simulink subsystem "AUVPlant"  (R2020a)
settings: Solver=VariableStepAuto  StartTime=0.0  StopTime=10.0  RelTol=1e-3
undefined symbols (not defined in the file or in its folder): dMaxX, dMaxY, dMinX, dMinY, dSeedX, dSeedY, dts, N, PWM, T200, tmax, tmin, waPhi, waPsi, waTheta, waX, waY, waZ, wfPhi, wfPsi, wfTheta, wfX, wfY, wfZ, wpPhi, wpPsi, wpTheta, wpX, wpY, wpZ
libraries: simulink x2
settings Model: Creator=lamarre  LastModifiedBy=lamarre

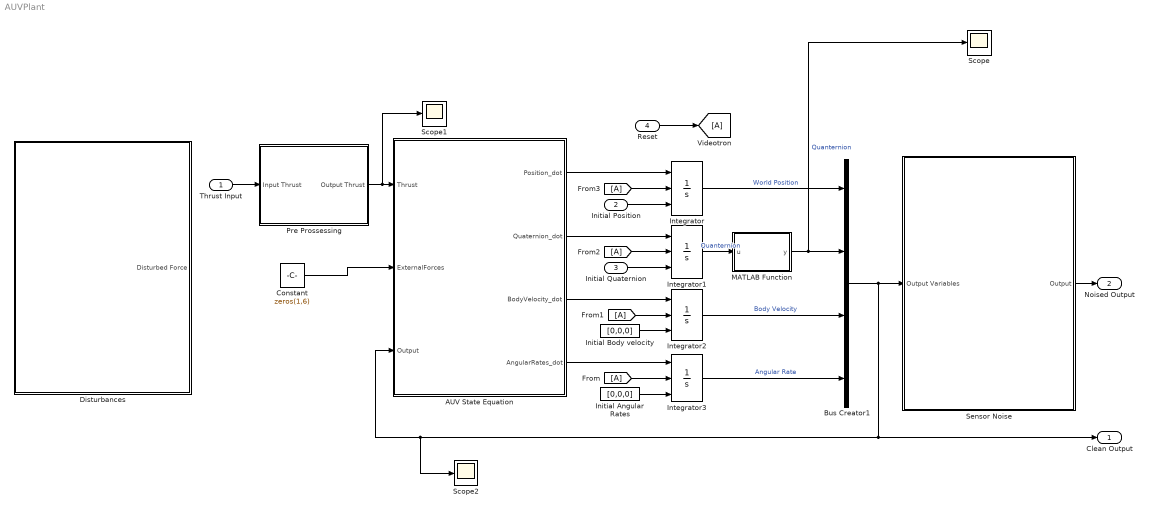
== system AUVPlant ==
  Thrust Input : Inport
  Initial Position : Inport  Port=2
  Initial Quaternion : Inport  Port=3
  Reset : Inport  Port=4
  AUV State Equation : MATLAB Function  TreatAsAtomicUnit=on  SystemSampleTime=.005
  Bus Creator1 : BusCreator  Inputs=4
  Constant : Constant  Value=zeros(1,6)
  Disturbances : Subsystem
  Initial Angular Rates : Constant  Value=[0,0,0]
  "Initial Body velocity " : Constant  Value=[0,0,0]
  Integrator : Integrator  ExternalReset=rising  InitialConditionSource=external  InitialCondition=[0,0,1]
  Integrator1 : Integrator  ExternalReset=rising  InitialConditionSource=external  InitialCondition=[1,0,0,0]
  Integrator2 : Integrator  ExternalReset=rising  InitialConditionSource=external  InitialCondition=[0,0,0]
  Integrator3 : Integrator  ExternalReset=rising  InitialConditionSource=external  InitialCondition=[0,0,0]
  MATLAB Function : MATLAB Function  TreatAsAtomicUnit=on
  Pre Prossessing : Subsystem
  Scope : Scope
  Scope1 : Scope
  Scope2 : Scope
  Sensor Noise : Subsystem
  Clean Output : Outport
  Noised Output : Outport  Port=2
  wires:
  "Initial Body velocity "/1 -> Integrator2/3
  AUV State Equation/2(Quaternion_dot) -> Integrator1/1
  Integrator/1 -> Bus Creator1/1  "World Position"
  Integrator2/1 -> Bus Creator1/3  "Body Velocity"
  AUV State Equation/1(Position_dot) -> Integrator/1
  Initial Angular Rates/1 -> Integrator3/3
  Thrust Input/1 -> Pre Prossessing/1(Input Thrust)
  AUV State Equation/4(AngularRates_dot) -> Integrator3/1
  Integrator3/1 -> Bus Creator1/4  "Angular Rate"
  Initial Quaternion/1 -> Integrator1/3
  AUV State Equation/3(BodyVelocity_dot) -> Integrator2/1
  [A] -> Integrator3/2
  [A] -> Integrator2/2
  [A] -> Integrator1/2
  [A] -> Integrator/2
  Initial Position/1 -> Integrator/3
  Reset/1 -> [A]
  Sensor Noise/1(Output) -> Noised Output/1
  Pre Prossessing/1(Output Thrust) -> AUV State Equation/1(Thrust), Scope1/1
  Bus Creator1/1 -> AUV State Equation/3(Output), Scope2/1, Clean Output/1, Sensor Noise/1(Output Variables)
  Integrator1/1 -> MATLAB Function/1(u)  "Quanternion"
  Constant/1 -> AUV State Equation/2(ExternalForces)
  MATLAB Function/1(y) -> Bus Creator1/2, Scope/1  "Quanternion"

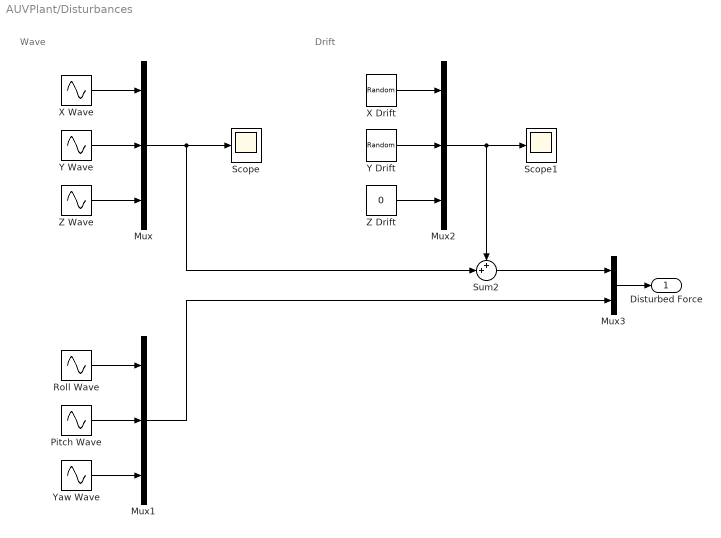
== system AUVPlant/Disturbances ==
  note: Drift
  note: Wave
  Mux : Mux  Inputs=3
  Mux1 : Mux  Inputs=3
  Mux2 : Mux  Inputs=3
  Mux3 : Mux  Inputs=2
  Pitch Wave : Sin  Amplitude=waTheta  Frequency=wfTheta  Phase=wpTheta  SampleTime=0
  Roll Wave : Sin  Amplitude=waPhi  Frequency=wfPhi  Phase=wpPhi  SampleTime=0
  Scope : Scope
  Scope1 : Scope
  Sum2 : Sum  Inputs=++|
  X Drift : UniformRandomNumber  Minimum=dMinX  Maximum=dMaxX  Seed=dSeedX  SampleTime=dts
  X Wave : Sin  Amplitude=waX  Frequency=wfX  Phase=wpX  SampleTime=0
  Y Drift : UniformRandomNumber  Minimum=dMinY  Maximum=dMaxY  Seed=dSeedY  SampleTime=dts
  Y Wave : Sin  Amplitude=waY  Frequency=wfY  Phase=wpY  SampleTime=0
  Yaw Wave : Sin  Amplitude=waPsi  Frequency=wfPsi  Phase=wpPsi  SampleTime=0
  Z Drift : Constant  Value=0
  Z Wave : Sin  Amplitude=waZ  Frequency=wfZ  Phase=wpZ  SampleTime=0
  Disturbed Force : Outport
  wires:
  Roll Wave/1 -> Mux1/1
  Pitch Wave/1 -> Mux1/2
  Mux3/1 -> Disturbed Force/1
  Sum2/1 -> Mux3/1
  X Wave/1 -> Mux/1
  Y Wave/1 -> Mux/2
  Z Wave/1 -> Mux/3
  Yaw Wave/1 -> Mux1/3
  Mux1/1 -> Mux3/2
  Mux2/1 -> Scope1/1, Sum2/1
  X Drift/1 -> Mux2/1
  Y Drift/1 -> Mux2/2
  Mux/1 -> Sum2/2, Scope/1
  Z Drift/1 -> Mux2/3

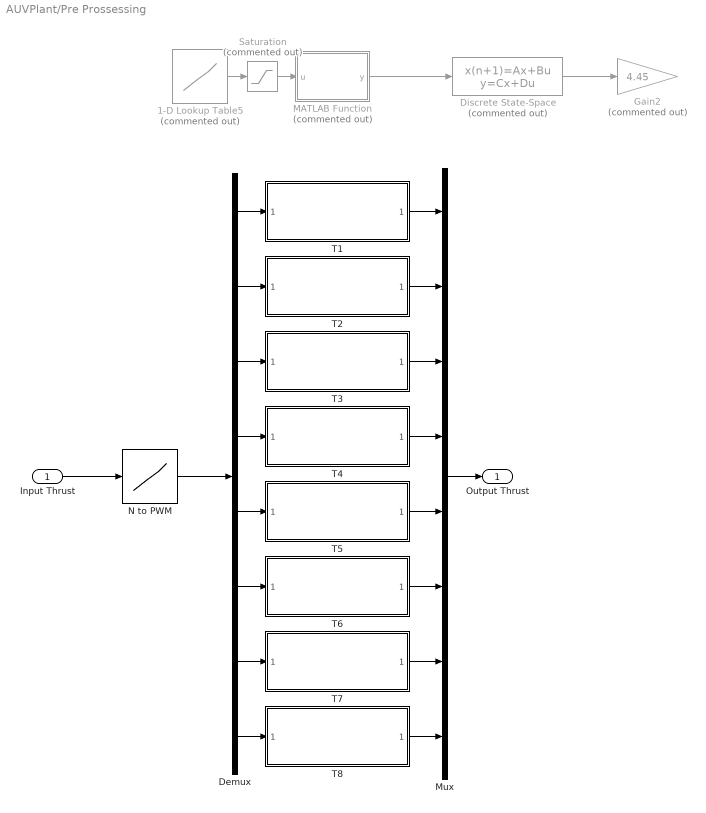
== system AUVPlant/Pre Prossessing ==
  Input Thrust : Inport
  1-D Lookup Table5 : Lookup_n-D  Commented=on  NumberOfTableDimensions=1  BreakpointsForDimension1=N  Table=PWM  InterpMethod=Nearest  InternalRulePriority=Speed  RndMeth=Simplest  InputSameDT=on
  Demux : Demux  Outputs=8
  Discrete State-Space : DiscreteStateSpace  Commented=on  A=T200.A  B=T200.B  C=T200.C  D=T200.D  SampleTime=T200.Ts
  Gain2 : Gain  Commented=on  Gain=4.45
  MATLAB Function : MATLAB Function  Commented=on  TreatAsAtomicUnit=on
  Mux : Mux  Inputs=8
  N to PWM : Lookup_n-D  NumberOfTableDimensions=1  BreakpointsForDimension1=PWM  Table=N  InterpMethod=Nearest  ExtrapMethod=Clip  InternalRulePriority=Speed  RndMeth=Simplest  InputSameDT=on
  Saturation : Saturate  Commented=on  UpperLimit=tmax  LowerLimit=tmin  LinearizeAsGain=off  ZeroCross=off
  T{1..8} (8 alike) : Subsystem  ReferencedSubsystem=ThrusterModel
  Output Thrust : Outport
  wires:
  Input Thrust/1 -> N to PWM/1
  N to PWM/1 -> Demux/1
  Saturation/1 -> MATLAB Function/1(u)
  1-D Lookup Table5/1 -> Saturation/1
  Discrete State-Space/1 -> Gain2/1
  MATLAB Function/1(y) -> Discrete State-Space/1
  Demux/1 -> T1/1
  Demux/2 -> T2/1
  Demux/3 -> T3/1
  Demux/4 -> T4/1
  Demux/5 -> T5/1
  Demux/6 -> T6/1
  Demux/8 -> T8/1
  Demux/7 -> T7/1
  T1/1 -> Mux/1
  T2/1 -> Mux/2
  T3/1 -> Mux/3
  T4/1 -> Mux/4
  T5/1 -> Mux/5
  T6/1 -> Mux/6
  T7/1 -> Mux/7
  T8/1 -> Mux/8
  Mux/1 -> Output Thrust/1

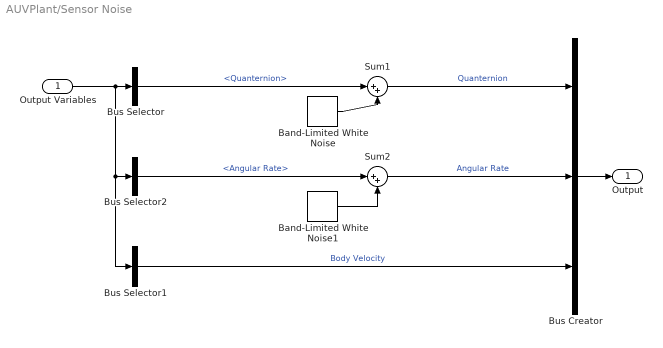
== system AUVPlant/Sensor Noise ==
  Output Variables : Inport
  Band-Limited White Noise : simulink/Sources/Band-Limited White Noise  Cov=[0.00000000025]  Ts=1/100  seed=[23341]
  Band-Limited White Noise1 : simulink/Sources/Band-Limited White Noise  Cov=[0.0000000004]  Ts=1/100  seed=[23341]
  Bus Creator : BusCreator  Inputs=3
  Bus Selector : BusSelector  OutputSignals=Quanternion
  Bus Selector1 : BusSelector  OutputSignals=Body Velocity  OutputAsBus=on
  Bus Selector2 : BusSelector  OutputSignals=Angular Rate
  Sum1 : Sum  Inputs=|++
  Sum2 : Sum  Inputs=|++
  Output : Outport
  wires:
  Sum2/1 -> Bus Creator/2  "Angular Rate"
  Sum1/1 -> Bus Creator/1  "Quanternion"
  Band-Limited White Noise1/1 -> Sum2/2
  Bus Selector2/1 -> Sum2/1  "<Angular Rate>"
  Bus Creator/1 -> Output/1
  Bus Selector1/1 -> Bus Creator/3  "Body Velocity"
  Bus Selector/1 -> Sum1/1  "<Quanternion>"
  Output Variables/1 -> Bus Selector/1, Bus Selector1/1, Bus Selector2/1
  Band-Limited White Noise/1 -> Sum1/2

== matlab function AUVPlant/MATLAB Function ==
  data: u input size=4; y output size=4
function y = Normalize(u)

d=norm(u);
y = u/d;

== matlab function AUVPlant/AUV State Equation ==
  data: Thrust input; ExternalForces input; Output input; Position_dot output size=3; Quaternion_dot output size=4; BodyVelocity_dot output size=3; AngularRates_dot output size=3
function [Position_dot,Quaternion_dot,BodyVelocity_dot, AngularRates_dot] = AUVStateEquation(Thrust,ExternalForces,Output)

Dynamics=AUVFossenSimFcn(Output,ExternalForces,Thrust);

Position_dot=Dynamics(1:3);
Quaternion_dot = Dynamics(4:7);
BodyVelocity_dot= Dynamics(8:10);
AngularRates_dot = Dynamics(11:13);

== matlab function AUVPlant/Pre Prossessing/MATLAB Function ==
  data: u input; y output
function y = fcn(u)
pwm=u-1500;
if pwm>=0 
    y=pwm;
else
   y=pwm*0.77969348659;
end
